simulink model "TST_RailP_PRV"  (R2016b)
settings: Solver=FixedStepDiscrete  StartTime=0.0  StopTime=simTime  FixedStep=sampleTime  RelTol=1e-3
values from neighbouring files (symbols this model uses):
  testCase = 1    [initTST_RailP_PRV_001.m]    (also in initTST_RailP_PRV_002.m = 2)
libraries: UnitTest_Lib x18, simulink x3
settings Model: Creator=liangyunbo  LastModifiedBy=liangyunbo
settings DebuggingCC: SignalRangeChecking=error

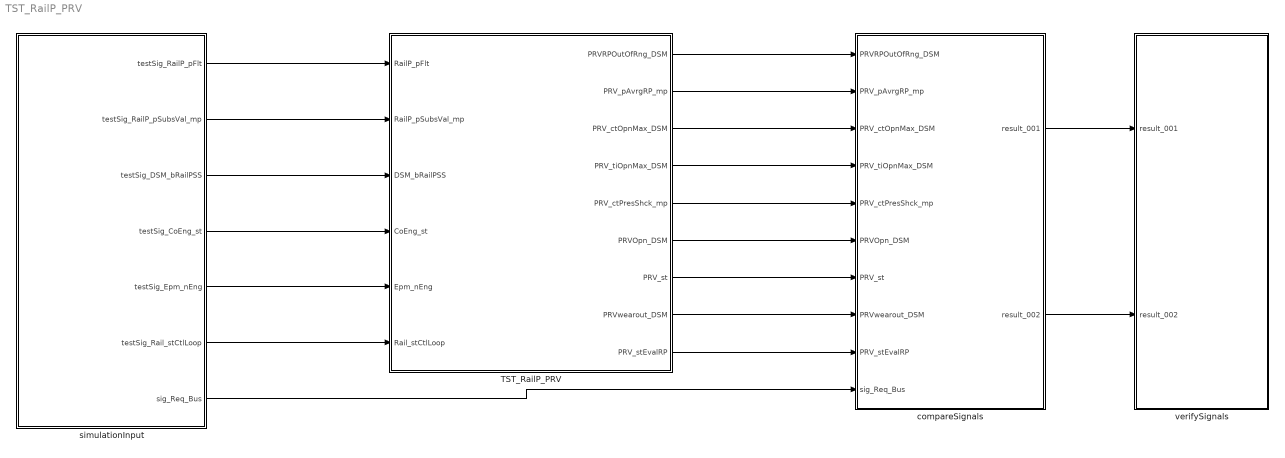
== system TST_RailP_PRV ==
  TST_RailP_PRV : Subsystem
  compareSignals : Subsystem
  simulationInput : Subsystem
  verifySignals : Subsystem
  wires:
  simulationInput/1(testSig_RailP_pFlt) -> TST_RailP_PRV/1(RailP_pFlt)
  simulationInput/2(testSig_RailP_pSubsVal_mp) -> TST_RailP_PRV/2(RailP_pSubsVal_mp)
  simulationInput/3(testSig_DSM_bRailPSS) -> TST_RailP_PRV/3(DSM_bRailPSS)
  simulationInput/4(testSig_CoEng_st) -> TST_RailP_PRV/4(CoEng_st)
  simulationInput/5(testSig_Epm_nEng) -> TST_RailP_PRV/5(Epm_nEng)
  simulationInput/6(testSig_Rail_stCtlLoop) -> TST_RailP_PRV/6(Rail_stCtlLoop)
  TST_RailP_PRV/1(PRVRPOutOfRng_DSM) -> compareSignals/1(PRVRPOutOfRng_DSM)
  TST_RailP_PRV/2(PRV_pAvrgRP_mp) -> compareSignals/2(PRV_pAvrgRP_mp)
  TST_RailP_PRV/3(PRV_ctOpnMax_DSM) -> compareSignals/3(PRV_ctOpnMax_DSM)
  TST_RailP_PRV/4(PRV_tiOpnMax_DSM) -> compareSignals/4(PRV_tiOpnMax_DSM)
  TST_RailP_PRV/5(PRV_ctPresShck_mp) -> compareSignals/5(PRV_ctPresShck_mp)
  TST_RailP_PRV/6(PRVOpn_DSM) -> compareSignals/6(PRVOpn_DSM)
  TST_RailP_PRV/7(PRV_st) -> compareSignals/7(PRV_st)
  TST_RailP_PRV/8(PRVwearout_DSM) -> compareSignals/8(PRVwearout_DSM)
  TST_RailP_PRV/9(PRV_stEvalRP) -> compareSignals/9(PRV_stEvalRP)
  simulationInput/7(sig_Req_Bus) -> compareSignals/10(sig_Req_Bus)
  compareSignals/1(result_001) -> verifySignals/1(result_001)
  compareSignals/2(result_002) -> verifySignals/2(result_002)

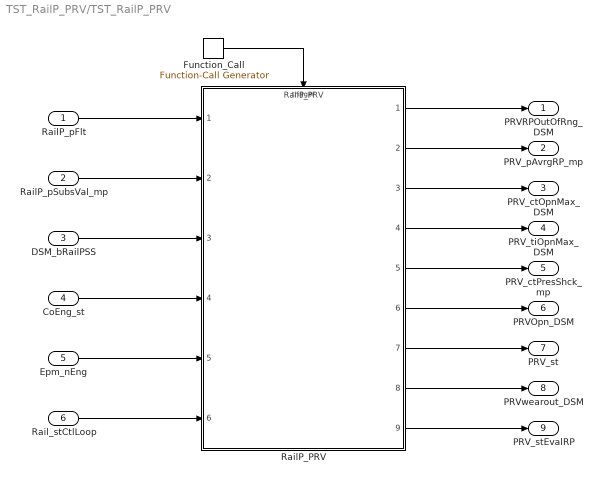
== system TST_RailP_PRV/TST_RailP_PRV ==
  RailP_pFlt : Inport
  RailP_pSubsVal_mp : Inport  Port=2
  DSM_bRailPSS : Inport  Port=3
  CoEng_st : Inport  Port=4
  Epm_nEng : Inport  Port=5
  Rail_stCtlLoop : Inport  Port=6
  Function_Call : simulink/Ports & Subsystems/Function-Call Generator  sample_time=sampleTime  numberOfIterations=1
  RailP_PRV : ModelReference  ModelNameDialog=RailP_PRV  SimulationMode=Normal  ModelReferenceVersion=1.208  TriggerPortName=function  TriggerPortTriggerType=function-call  TriggerPortStatesWhenEnabling=held
  PRVRPOutOfRng_DSM : Outport
  PRV_pAvrgRP_mp : Outport  Port=2
  PRV_ctOpnMax_DSM : Outport  Port=3
  PRV_tiOpnMax_DSM : Outport  Port=4
  PRV_ctPresShck_mp : Outport  Port=5
  PRVOpn_DSM : Outport  Port=6
  PRV_st : Outport  Port=7
  PRVwearout_DSM : Outport  Port=8
  PRV_stEvalRP : Outport  Port=9
  wires:
  Function_Call/1 -> RailP_PRV/Trigger
  RailP_pFlt/1 -> RailP_PRV/1
  RailP_pSubsVal_mp/1 -> RailP_PRV/2
  DSM_bRailPSS/1 -> RailP_PRV/3
  CoEng_st/1 -> RailP_PRV/4
  Epm_nEng/1 -> RailP_PRV/5
  Rail_stCtlLoop/1 -> RailP_PRV/6
  RailP_PRV/1 -> PRVRPOutOfRng_DSM/1
  RailP_PRV/2 -> PRV_pAvrgRP_mp/1
  RailP_PRV/3 -> PRV_ctOpnMax_DSM/1
  RailP_PRV/4 -> PRV_tiOpnMax_DSM/1
  RailP_PRV/5 -> PRV_ctPresShck_mp/1
  RailP_PRV/6 -> PRVOpn_DSM/1
  RailP_PRV/7 -> PRV_st/1
  RailP_PRV/8 -> PRVwearout_DSM/1
  RailP_PRV/9 -> PRV_stEvalRP/1

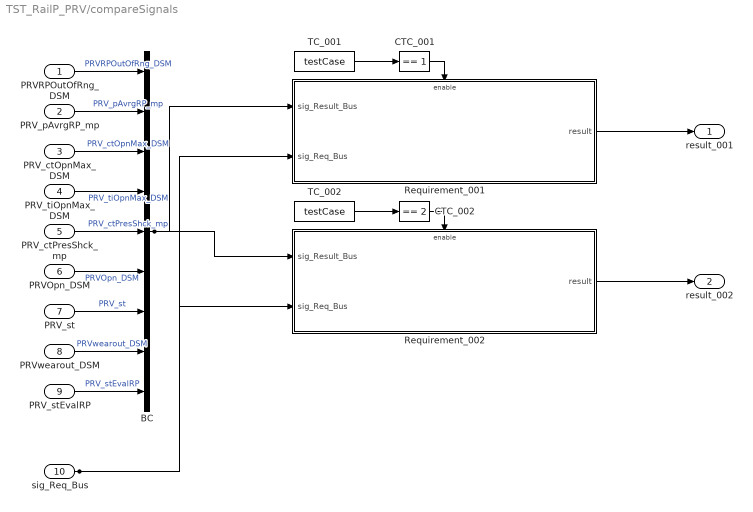
== system TST_RailP_PRV/compareSignals ==
  PRVRPOutOfRng_DSM : Inport
  PRV_pAvrgRP_mp : Inport  Port=2
  PRV_ctOpnMax_DSM : Inport  Port=3
  PRV_tiOpnMax_DSM : Inport  Port=4
  PRV_ctPresShck_mp : Inport  Port=5
  PRVOpn_DSM : Inport  Port=6
  PRV_st : Inport  Port=7
  PRVwearout_DSM : Inport  Port=8
  PRV_stEvalRP : Inport  Port=9
  sig_Req_Bus : Inport  Port=10
  BC : BusCreator  Inputs=9
  CTC_001 : simulink/Logic and Bit Operations/Compare To Constant  relop===  const=1  OutDataTypeStr=boolean
  CTC_002 : simulink/Logic and Bit Operations/Compare To Constant  relop===  const=2  OutDataTypeStr=boolean
  Requirement_001 : Subsystem
  Requirement_002 : Subsystem
  TC_001 : Constant  Value=testCase
  TC_002 : Constant  Value=testCase
  result_001 : Outport
  result_002 : Outport  Port=2
  wires:
  PRVRPOutOfRng_DSM/1 -> BC/1  "PRVRPOutOfRng_DSM"
  PRV_pAvrgRP_mp/1 -> BC/2  "PRV_pAvrgRP_mp"
  PRV_ctOpnMax_DSM/1 -> BC/3  "PRV_ctOpnMax_DSM"
  PRV_tiOpnMax_DSM/1 -> BC/4  "PRV_tiOpnMax_DSM"
  PRV_ctPresShck_mp/1 -> BC/5  "PRV_ctPresShck_mp"
  PRVOpn_DSM/1 -> BC/6  "PRVOpn_DSM"
  PRV_st/1 -> BC/7  "PRV_st"
  PRVwearout_DSM/1 -> BC/8  "PRVwearout_DSM"
  PRV_stEvalRP/1 -> BC/9  "PRV_stEvalRP"
  TC_001/1 -> CTC_001/1
  CTC_001/1 -> Requirement_001/Enable
  sig_Req_Bus/1 -> Requirement_001/2(sig_Req_Bus), Requirement_002/2(sig_Req_Bus)
  BC/1 -> Requirement_001/1(sig_Result_Bus), Requirement_002/1(sig_Result_Bus)
  Requirement_001/1(result) -> result_001/1
  TC_002/1 -> CTC_002/1
  CTC_002/1 -> Requirement_002/Enable
  Requirement_002/1(result) -> result_002/1

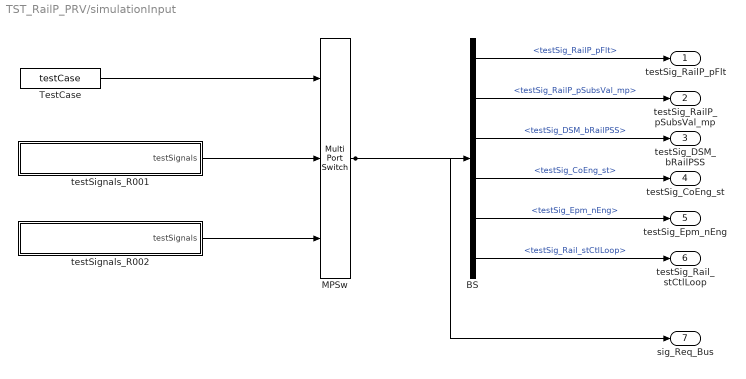
== system TST_RailP_PRV/simulationInput ==
  BS : BusSelector  OutputSignals=testSig_RailP_pFlt,testSig_RailP_pSubsVal_mp,testSig_DSM_bRailPSS,testSig_CoEng_st,testSig_Epm_nEng,testSig_Rail_stCtlLoop
  MPSw : MultiPortSwitch  Inputs=2  SaturateOnIntegerOverflow=on  InputSameDT=on
  TestCase : Constant  Value=testCase
  testSignals_R001 : Subsystem
  testSignals_R002 : Subsystem
  testSig_RailP_pFlt : Outport
  testSig_RailP_pSubsVal_mp : Outport  Port=2
  testSig_DSM_bRailPSS : Outport  Port=3
  testSig_CoEng_st : Outport  Port=4
  testSig_Epm_nEng : Outport  Port=5
  testSig_Rail_stCtlLoop : Outport  Port=6
  sig_Req_Bus : Outport  Port=7
  wires:
  BS/1 -> testSig_RailP_pFlt/1  "<testSig_RailP_pFlt>"
  BS/2 -> testSig_RailP_pSubsVal_mp/1  "<testSig_RailP_pSubsVal_mp>"
  BS/3 -> testSig_DSM_bRailPSS/1  "<testSig_DSM_bRailPSS>"
  BS/4 -> testSig_CoEng_st/1  "<testSig_CoEng_st>"
  BS/5 -> testSig_Epm_nEng/1  "<testSig_Epm_nEng>"
  BS/6 -> testSig_Rail_stCtlLoop/1  "<testSig_Rail_stCtlLoop>"
  MPSw/1 -> BS/1, sig_Req_Bus/1
  TestCase/1 -> MPSw/1
  testSignals_R001/1(testSignals) -> MPSw/2
  testSignals_R002/1(testSignals) -> MPSw/3

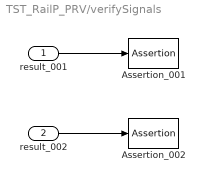
== system TST_RailP_PRV/verifySignals ==
  result_001 : Inport
  result_002 : Inport  Port=2
  Assertion_001 : Assertion  Enabled=off
  Assertion_002 : Assertion  Enabled=off
  wires:
  result_001/1 -> Assertion_001/1
  result_002/1 -> Assertion_002/1

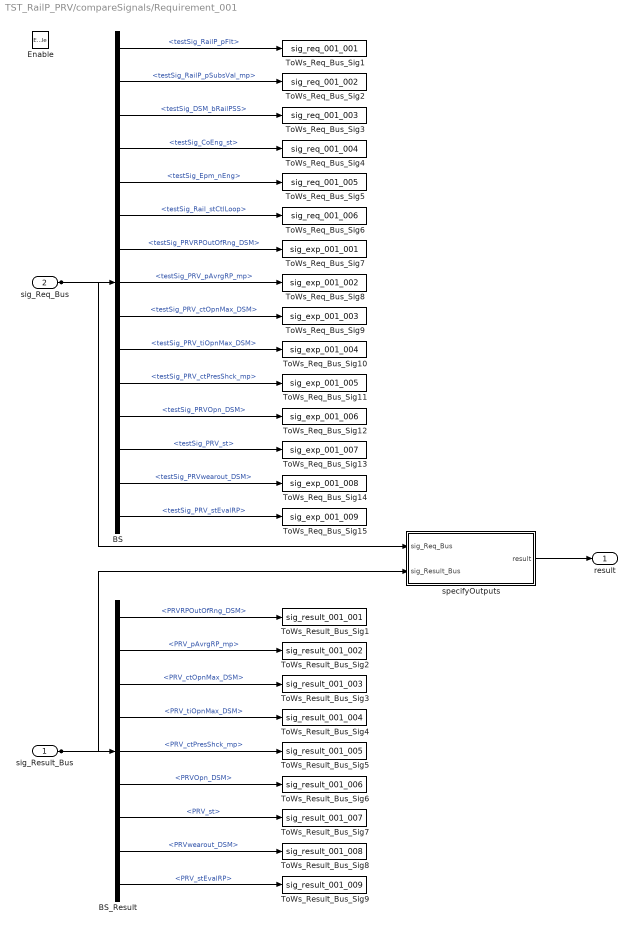
== system TST_RailP_PRV/compareSignals/Requirement_001 ==
  sig_Result_Bus : Inport
  sig_Req_Bus : Inport  Port=2
  Enable : EnablePort
  BS : BusSelector  OutputSignals=testSig_RailP_pFlt,testSig_RailP_pSubsVal_mp,testSig_DSM_bRailPSS,testSig_CoEng_st,testSig_Epm_nEng,testSig_Rail_stCtlLoop,testSig_PRVRPOutOfRng_DSM,testSig_PRV_pAvrgRP_mp,testSig_PRV_ctOpnMax_DSM,testSig_PRV_tiOpnMax_DSM,testSig_PRV_ctPresShck_mp,testSig_PRVOpn_DSM,testSig_PRV_st,testSig_PRVwearout_DSM,testSig_PRV_stEvalRP
  BS_Result : BusSelector  OutputSignals=PRVRPOutOfRng_DSM,PRV_pAvrgRP_mp,PRV_ctOpnMax_DSM,PRV_tiOpnMax_DSM,PRV_ctPresShck_mp,PRVOpn_DSM,PRV_st,PRVwearout_DSM,PRV_stEvalRP
  ToWs_Req_Bus_Sig1 : ToWorkspace  VariableName=sig_req_001_001  SaveFormat=Structure With Time
  ToWs_Req_Bus_Sig10 : ToWorkspace  VariableName=sig_exp_001_004  SaveFormat=Structure With Time
  ToWs_Req_Bus_Sig11 : ToWorkspace  VariableName=sig_exp_001_005  SaveFormat=Structure With Time
  ToWs_Req_Bus_Sig12 : ToWorkspace  VariableName=sig_exp_001_006  SaveFormat=Structure With Time
  ToWs_Req_Bus_Sig13 : ToWorkspace  VariableName=sig_exp_001_007  SaveFormat=Structure With Time
  ToWs_Req_Bus_Sig14 : ToWorkspace  VariableName=sig_exp_001_008  SaveFormat=Structure With Time
  ToWs_Req_Bus_Sig15 : ToWorkspace  VariableName=sig_exp_001_009  SaveFormat=Structure With Time
  ToWs_Req_Bus_Sig2 : ToWorkspace  VariableName=sig_req_001_002  SaveFormat=Structure With Time
  ToWs_Req_Bus_Sig3 : ToWorkspace  VariableName=sig_req_001_003  SaveFormat=Structure With Time
  ToWs_Req_Bus_Sig4 : ToWorkspace  VariableName=sig_req_001_004  SaveFormat=Structure With Time
  ToWs_Req_Bus_Sig5 : ToWorkspace  VariableName=sig_req_001_005  SaveFormat=Structure With Time
  ToWs_Req_Bus_Sig6 : ToWorkspace  VariableName=sig_req_001_006  SaveFormat=Structure With Time
  ToWs_Req_Bus_Sig7 : ToWorkspace  VariableName=sig_exp_001_001  SaveFormat=Structure With Time
  ToWs_Req_Bus_Sig8 : ToWorkspace  VariableName=sig_exp_001_002  SaveFormat=Structure With Time
  ToWs_Req_Bus_Sig9 : ToWorkspace  VariableName=sig_exp_001_003  SaveFormat=Structure With Time
  ToWs_Result_Bus_Sig1 : ToWorkspace  VariableName=sig_result_001_001  SaveFormat=Structure With Time
  ToWs_Result_Bus_Sig2 : ToWorkspace  VariableName=sig_result_001_002  SaveFormat=Structure With Time
  ToWs_Result_Bus_Sig3 : ToWorkspace  VariableName=sig_result_001_003  SaveFormat=Structure With Time
  ToWs_Result_Bus_Sig4 : ToWorkspace  VariableName=sig_result_001_004  SaveFormat=Structure With Time
  ToWs_Result_Bus_Sig5 : ToWorkspace  VariableName=sig_result_001_005  SaveFormat=Structure With Time
  ToWs_Result_Bus_Sig6 : ToWorkspace  VariableName=sig_result_001_006  SaveFormat=Structure With Time
  ToWs_Result_Bus_Sig7 : ToWorkspace  VariableName=sig_result_001_007  SaveFormat=Structure With Time
  ToWs_Result_Bus_Sig8 : ToWorkspace  VariableName=sig_result_001_008  SaveFormat=Structure With Time
  ToWs_Result_Bus_Sig9 : ToWorkspace  VariableName=sig_result_001_009  SaveFormat=Structure With Time
  specifyOutputs : Subsystem
  result : Outport
  wires:
  sig_Req_Bus/1 -> BS/1, specifyOutputs/1(sig_Req_Bus)
  BS/1 -> ToWs_Req_Bus_Sig1/1  "<testSig_RailP_pFlt>"
  BS/2 -> ToWs_Req_Bus_Sig2/1  "<testSig_RailP_pSubsVal_mp>"
  BS/3 -> ToWs_Req_Bus_Sig3/1  "<testSig_DSM_bRailPSS>"
  BS/4 -> ToWs_Req_Bus_Sig4/1  "<testSig_CoEng_st>"
  BS/5 -> ToWs_Req_Bus_Sig5/1  "<testSig_Epm_nEng>"
  BS/6 -> ToWs_Req_Bus_Sig6/1  "<testSig_Rail_stCtlLoop>"
  BS/7 -> ToWs_Req_Bus_Sig7/1  "<testSig_PRVRPOutOfRng_DSM>"
  BS/8 -> ToWs_Req_Bus_Sig8/1  "<testSig_PRV_pAvrgRP_mp>"
  BS/9 -> ToWs_Req_Bus_Sig9/1  "<testSig_PRV_ctOpnMax_DSM>"
  BS/10 -> ToWs_Req_Bus_Sig10/1  "<testSig_PRV_tiOpnMax_DSM>"
  BS/11 -> ToWs_Req_Bus_Sig11/1  "<testSig_PRV_ctPresShck_mp>"
  BS/12 -> ToWs_Req_Bus_Sig12/1  "<testSig_PRVOpn_DSM>"
  BS/13 -> ToWs_Req_Bus_Sig13/1  "<testSig_PRV_st>"
  BS/14 -> ToWs_Req_Bus_Sig14/1  "<testSig_PRVwearout_DSM>"
  BS/15 -> ToWs_Req_Bus_Sig15/1  "<testSig_PRV_stEvalRP>"
  sig_Result_Bus/1 -> BS_Result/1, specifyOutputs/2(sig_Result_Bus)
  BS_Result/1 -> ToWs_Result_Bus_Sig1/1  "<PRVRPOutOfRng_DSM>"
  BS_Result/2 -> ToWs_Result_Bus_Sig2/1  "<PRV_pAvrgRP_mp>"
  BS_Result/3 -> ToWs_Result_Bus_Sig3/1  "<PRV_ctOpnMax_DSM>"
  BS_Result/4 -> ToWs_Result_Bus_Sig4/1  "<PRV_tiOpnMax_DSM>"
  BS_Result/5 -> ToWs_Result_Bus_Sig5/1  "<PRV_ctPresShck_mp>"
  BS_Result/6 -> ToWs_Result_Bus_Sig6/1  "<PRVOpn_DSM>"
  BS_Result/7 -> ToWs_Result_Bus_Sig7/1  "<PRV_st>"
  BS_Result/8 -> ToWs_Result_Bus_Sig8/1  "<PRVwearout_DSM>"
  BS_Result/9 -> ToWs_Result_Bus_Sig9/1  "<PRV_stEvalRP>"
  specifyOutputs/1(result) -> result/1

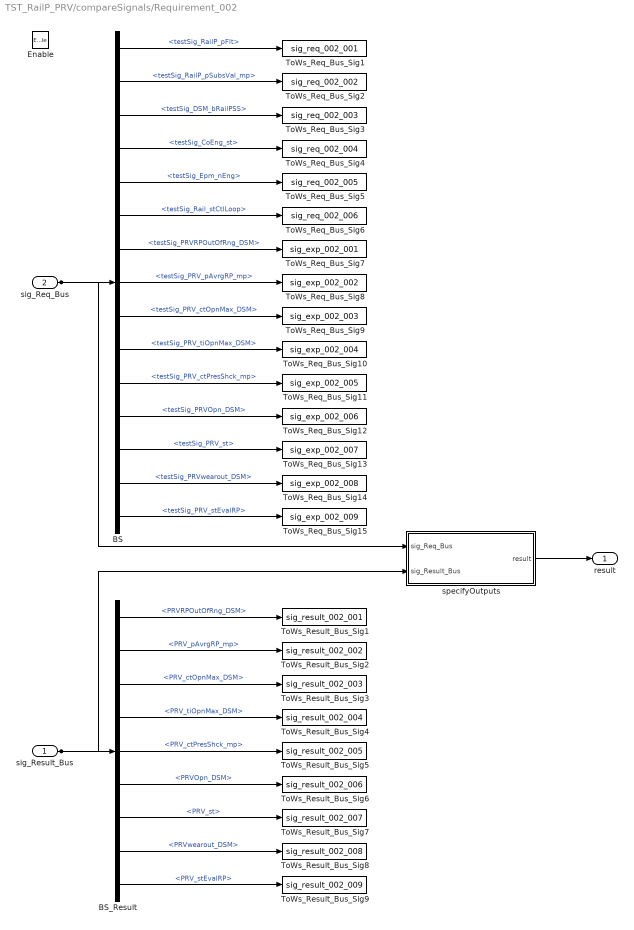
== system TST_RailP_PRV/compareSignals/Requirement_002 ==
  sig_Result_Bus : Inport
  sig_Req_Bus : Inport  Port=2
  Enable : EnablePort
  BS : BusSelector  OutputSignals=testSig_RailP_pFlt,testSig_RailP_pSubsVal_mp,testSig_DSM_bRailPSS,testSig_CoEng_st,testSig_Epm_nEng,testSig_Rail_stCtlLoop,testSig_PRVRPOutOfRng_DSM,testSig_PRV_pAvrgRP_mp,testSig_PRV_ctOpnMax_DSM,testSig_PRV_tiOpnMax_DSM,testSig_PRV_ctPresShck_mp,testSig_PRVOpn_DSM,testSig_PRV_st,testSig_PRVwearout_DSM,testSig_PRV_stEvalRP
  BS_Result : BusSelector  OutputSignals=PRVRPOutOfRng_DSM,PRV_pAvrgRP_mp,PRV_ctOpnMax_DSM,PRV_tiOpnMax_DSM,PRV_ctPresShck_mp,PRVOpn_DSM,PRV_st,PRVwearout_DSM,PRV_stEvalRP
  ToWs_Req_Bus_Sig1 : ToWorkspace  VariableName=sig_req_002_001  SaveFormat=Structure With Time
  ToWs_Req_Bus_Sig10 : ToWorkspace  VariableName=sig_exp_002_004  SaveFormat=Structure With Time
  ToWs_Req_Bus_Sig11 : ToWorkspace  VariableName=sig_exp_002_005  SaveFormat=Structure With Time
  ToWs_Req_Bus_Sig12 : ToWorkspace  VariableName=sig_exp_002_006  SaveFormat=Structure With Time
  ToWs_Req_Bus_Sig13 : ToWorkspace  VariableName=sig_exp_002_007  SaveFormat=Structure With Time
  ToWs_Req_Bus_Sig14 : ToWorkspace  VariableName=sig_exp_002_008  SaveFormat=Structure With Time
  ToWs_Req_Bus_Sig15 : ToWorkspace  VariableName=sig_exp_002_009  SaveFormat=Structure With Time
  ToWs_Req_Bus_Sig2 : ToWorkspace  VariableName=sig_req_002_002  SaveFormat=Structure With Time
  ToWs_Req_Bus_Sig3 : ToWorkspace  VariableName=sig_req_002_003  SaveFormat=Structure With Time
  ToWs_Req_Bus_Sig4 : ToWorkspace  VariableName=sig_req_002_004  SaveFormat=Structure With Time
  ToWs_Req_Bus_Sig5 : ToWorkspace  VariableName=sig_req_002_005  SaveFormat=Structure With Time
  ToWs_Req_Bus_Sig6 : ToWorkspace  VariableName=sig_req_002_006  SaveFormat=Structure With Time
  ToWs_Req_Bus_Sig7 : ToWorkspace  VariableName=sig_exp_002_001  SaveFormat=Structure With Time
  ToWs_Req_Bus_Sig8 : ToWorkspace  VariableName=sig_exp_002_002  SaveFormat=Structure With Time
  ToWs_Req_Bus_Sig9 : ToWorkspace  VariableName=sig_exp_002_003  SaveFormat=Structure With Time
  ToWs_Result_Bus_Sig1 : ToWorkspace  VariableName=sig_result_002_001  SaveFormat=Structure With Time
  ToWs_Result_Bus_Sig2 : ToWorkspace  VariableName=sig_result_002_002  SaveFormat=Structure With Time
  ToWs_Result_Bus_Sig3 : ToWorkspace  VariableName=sig_result_002_003  SaveFormat=Structure With Time
  ToWs_Result_Bus_Sig4 : ToWorkspace  VariableName=sig_result_002_004  SaveFormat=Structure With Time
  ToWs_Result_Bus_Sig5 : ToWorkspace  VariableName=sig_result_002_005  SaveFormat=Structure With Time
  ToWs_Result_Bus_Sig6 : ToWorkspace  VariableName=sig_result_002_006  SaveFormat=Structure With Time
  ToWs_Result_Bus_Sig7 : ToWorkspace  VariableName=sig_result_002_007  SaveFormat=Structure With Time
  ToWs_Result_Bus_Sig8 : ToWorkspace  VariableName=sig_result_002_008  SaveFormat=Structure With Time
  ToWs_Result_Bus_Sig9 : ToWorkspace  VariableName=sig_result_002_009  SaveFormat=Structure With Time
  specifyOutputs : Subsystem
  result : Outport
  wires:
  sig_Req_Bus/1 -> BS/1, specifyOutputs/1(sig_Req_Bus)
  BS/1 -> ToWs_Req_Bus_Sig1/1  "<testSig_RailP_pFlt>"
  BS/2 -> ToWs_Req_Bus_Sig2/1  "<testSig_RailP_pSubsVal_mp>"
  BS/3 -> ToWs_Req_Bus_Sig3/1  "<testSig_DSM_bRailPSS>"
  BS/4 -> ToWs_Req_Bus_Sig4/1  "<testSig_CoEng_st>"
  BS/5 -> ToWs_Req_Bus_Sig5/1  "<testSig_Epm_nEng>"
  BS/6 -> ToWs_Req_Bus_Sig6/1  "<testSig_Rail_stCtlLoop>"
  BS/7 -> ToWs_Req_Bus_Sig7/1  "<testSig_PRVRPOutOfRng_DSM>"
  BS/8 -> ToWs_Req_Bus_Sig8/1  "<testSig_PRV_pAvrgRP_mp>"
  BS/9 -> ToWs_Req_Bus_Sig9/1  "<testSig_PRV_ctOpnMax_DSM>"
  BS/10 -> ToWs_Req_Bus_Sig10/1  "<testSig_PRV_tiOpnMax_DSM>"
  BS/11 -> ToWs_Req_Bus_Sig11/1  "<testSig_PRV_ctPresShck_mp>"
  BS/12 -> ToWs_Req_Bus_Sig12/1  "<testSig_PRVOpn_DSM>"
  BS/13 -> ToWs_Req_Bus_Sig13/1  "<testSig_PRV_st>"
  BS/14 -> ToWs_Req_Bus_Sig14/1  "<testSig_PRVwearout_DSM>"
  BS/15 -> ToWs_Req_Bus_Sig15/1  "<testSig_PRV_stEvalRP>"
  sig_Result_Bus/1 -> BS_Result/1, specifyOutputs/2(sig_Result_Bus)
  BS_Result/1 -> ToWs_Result_Bus_Sig1/1  "<PRVRPOutOfRng_DSM>"
  BS_Result/2 -> ToWs_Result_Bus_Sig2/1  "<PRV_pAvrgRP_mp>"
  BS_Result/3 -> ToWs_Result_Bus_Sig3/1  "<PRV_ctOpnMax_DSM>"
  BS_Result/4 -> ToWs_Result_Bus_Sig4/1  "<PRV_tiOpnMax_DSM>"
  BS_Result/5 -> ToWs_Result_Bus_Sig5/1  "<PRV_ctPresShck_mp>"
  BS_Result/6 -> ToWs_Result_Bus_Sig6/1  "<PRVOpn_DSM>"
  BS_Result/7 -> ToWs_Result_Bus_Sig7/1  "<PRV_st>"
  BS_Result/8 -> ToWs_Result_Bus_Sig8/1  "<PRVwearout_DSM>"
  BS_Result/9 -> ToWs_Result_Bus_Sig9/1  "<PRV_stEvalRP>"
  specifyOutputs/1(result) -> result/1

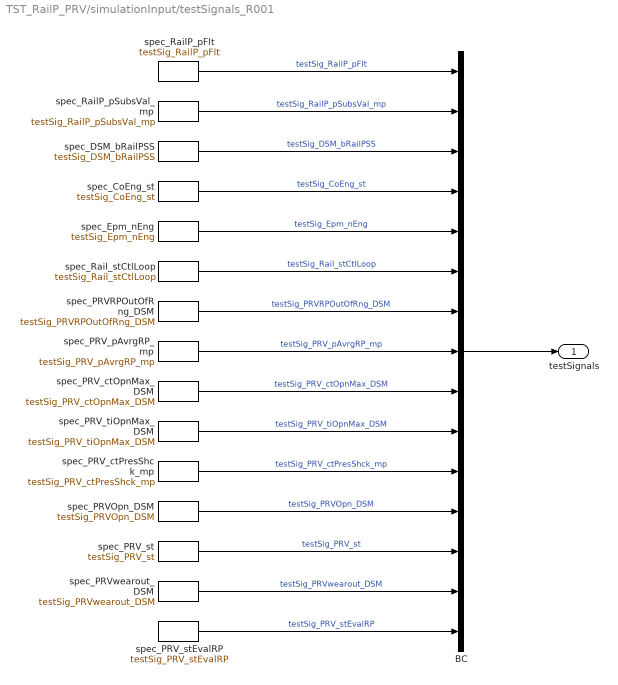
== system TST_RailP_PRV/simulationInput/testSignals_R001 ==
  BC : BusCreator  Inputs=15
  spec_CoEng_st : FromWorkspace  VariableName=testSig_CoEng_st  Interpolate=off  OutputAfterFinalValue=Holding final value
  spec_DSM_bRailPSS : FromWorkspace  VariableName=testSig_DSM_bRailPSS  Interpolate=off  OutputAfterFinalValue=Holding final value
  spec_Epm_nEng : FromWorkspace  VariableName=testSig_Epm_nEng  Interpolate=off  OutputAfterFinalValue=Holding final value
  spec_PRVOpn_DSM : FromWorkspace  VariableName=testSig_PRVOpn_DSM  Interpolate=off  OutputAfterFinalValue=Holding final value
  spec_PRVRPOutOfRng_DSM : FromWorkspace  VariableName=testSig_PRVRPOutOfRng_DSM  Interpolate=off  OutputAfterFinalValue=Holding final value
  spec_PRV_ctOpnMax_DSM : FromWorkspace  VariableName=testSig_PRV_ctOpnMax_DSM  Interpolate=off  OutputAfterFinalValue=Holding final value
  spec_PRV_ctPresShck_mp : FromWorkspace  VariableName=testSig_PRV_ctPresShck_mp  Interpolate=off  OutputAfterFinalValue=Holding final value
  spec_PRV_pAvrgRP_mp : FromWorkspace  VariableName=testSig_PRV_pAvrgRP_mp  Interpolate=off  OutputAfterFinalValue=Holding final value
  spec_PRV_st : FromWorkspace  VariableName=testSig_PRV_st  Interpolate=off  OutputAfterFinalValue=Holding final value
  spec_PRV_stEvalRP : FromWorkspace  VariableName=testSig_PRV_stEvalRP  Interpolate=off  OutputAfterFinalValue=Holding final value
  spec_PRV_tiOpnMax_DSM : FromWorkspace  VariableName=testSig_PRV_tiOpnMax_DSM  Interpolate=off  OutputAfterFinalValue=Holding final value
  spec_PRVwearout_DSM : FromWorkspace  VariableName=testSig_PRVwearout_DSM  Interpolate=off  OutputAfterFinalValue=Holding final value
  spec_RailP_pFlt : FromWorkspace  VariableName=testSig_RailP_pFlt  Interpolate=off  OutputAfterFinalValue=Holding final value
  spec_RailP_pSubsVal_mp : FromWorkspace  VariableName=testSig_RailP_pSubsVal_mp  Interpolate=off  OutputAfterFinalValue=Holding final value
  spec_Rail_stCtlLoop : FromWorkspace  VariableName=testSig_Rail_stCtlLoop  Interpolate=off  OutputAfterFinalValue=Holding final value
  testSignals : Outport
  wires:
  BC/1 -> testSignals/1
  spec_RailP_pFlt/1 -> BC/1  "testSig_RailP_pFlt"
  spec_RailP_pSubsVal_mp/1 -> BC/2  "testSig_RailP_pSubsVal_mp"
  spec_DSM_bRailPSS/1 -> BC/3  "testSig_DSM_bRailPSS"
  spec_CoEng_st/1 -> BC/4  "testSig_CoEng_st"
  spec_Epm_nEng/1 -> BC/5  "testSig_Epm_nEng"
  spec_Rail_stCtlLoop/1 -> BC/6  "testSig_Rail_stCtlLoop"
  spec_PRVRPOutOfRng_DSM/1 -> BC/7  "testSig_PRVRPOutOfRng_DSM"
  spec_PRV_pAvrgRP_mp/1 -> BC/8  "testSig_PRV_pAvrgRP_mp"
  spec_PRV_ctOpnMax_DSM/1 -> BC/9  "testSig_PRV_ctOpnMax_DSM"
  spec_PRV_tiOpnMax_DSM/1 -> BC/10  "testSig_PRV_tiOpnMax_DSM"
  spec_PRV_ctPresShck_mp/1 -> BC/11  "testSig_PRV_ctPresShck_mp"
  spec_PRVOpn_DSM/1 -> BC/12  "testSig_PRVOpn_DSM"
  spec_PRV_st/1 -> BC/13  "testSig_PRV_st"
  spec_PRVwearout_DSM/1 -> BC/14  "testSig_PRVwearout_DSM"
  spec_PRV_stEvalRP/1 -> BC/15  "testSig_PRV_stEvalRP"

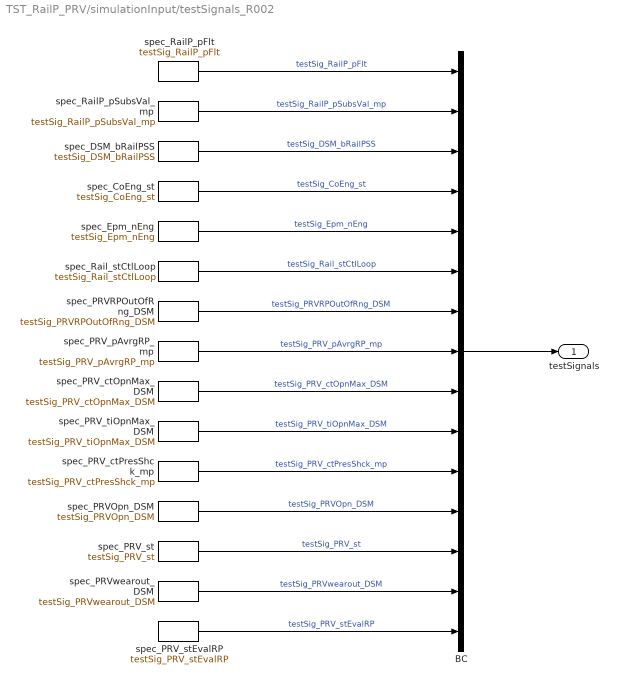
== system TST_RailP_PRV/simulationInput/testSignals_R002 ==
  BC : BusCreator  Inputs=15
  spec_CoEng_st : FromWorkspace  VariableName=testSig_CoEng_st  Interpolate=off  OutputAfterFinalValue=Holding final value
  spec_DSM_bRailPSS : FromWorkspace  VariableName=testSig_DSM_bRailPSS  Interpolate=off  OutputAfterFinalValue=Holding final value
  spec_Epm_nEng : FromWorkspace  VariableName=testSig_Epm_nEng  Interpolate=off  OutputAfterFinalValue=Holding final value
  spec_PRVOpn_DSM : FromWorkspace  VariableName=testSig_PRVOpn_DSM  Interpolate=off  OutputAfterFinalValue=Holding final value
  spec_PRVRPOutOfRng_DSM : FromWorkspace  VariableName=testSig_PRVRPOutOfRng_DSM  Interpolate=off  OutputAfterFinalValue=Holding final value
  spec_PRV_ctOpnMax_DSM : FromWorkspace  VariableName=testSig_PRV_ctOpnMax_DSM  Interpolate=off  OutputAfterFinalValue=Holding final value
  spec_PRV_ctPresShck_mp : FromWorkspace  VariableName=testSig_PRV_ctPresShck_mp  Interpolate=off  OutputAfterFinalValue=Holding final value
  spec_PRV_pAvrgRP_mp : FromWorkspace  VariableName=testSig_PRV_pAvrgRP_mp  Interpolate=off  OutputAfterFinalValue=Holding final value
  spec_PRV_st : FromWorkspace  VariableName=testSig_PRV_st  Interpolate=off  OutputAfterFinalValue=Holding final value
  spec_PRV_stEvalRP : FromWorkspace  VariableName=testSig_PRV_stEvalRP  Interpolate=off  OutputAfterFinalValue=Holding final value
  spec_PRV_tiOpnMax_DSM : FromWorkspace  VariableName=testSig_PRV_tiOpnMax_DSM  Interpolate=off  OutputAfterFinalValue=Holding final value
  spec_PRVwearout_DSM : FromWorkspace  VariableName=testSig_PRVwearout_DSM  Interpolate=off  OutputAfterFinalValue=Holding final value
  spec_RailP_pFlt : FromWorkspace  VariableName=testSig_RailP_pFlt  Interpolate=off  OutputAfterFinalValue=Holding final value
  spec_RailP_pSubsVal_mp : FromWorkspace  VariableName=testSig_RailP_pSubsVal_mp  Interpolate=off  OutputAfterFinalValue=Holding final value
  spec_Rail_stCtlLoop : FromWorkspace  VariableName=testSig_Rail_stCtlLoop  Interpolate=off  OutputAfterFinalValue=Holding final value
  testSignals : Outport
  wires:
  BC/1 -> testSignals/1
  spec_RailP_pFlt/1 -> BC/1  "testSig_RailP_pFlt"
  spec_RailP_pSubsVal_mp/1 -> BC/2  "testSig_RailP_pSubsVal_mp"
  spec_DSM_bRailPSS/1 -> BC/3  "testSig_DSM_bRailPSS"
  spec_CoEng_st/1 -> BC/4  "testSig_CoEng_st"
  spec_Epm_nEng/1 -> BC/5  "testSig_Epm_nEng"
  spec_Rail_stCtlLoop/1 -> BC/6  "testSig_Rail_stCtlLoop"
  spec_PRVRPOutOfRng_DSM/1 -> BC/7  "testSig_PRVRPOutOfRng_DSM"
  spec_PRV_pAvrgRP_mp/1 -> BC/8  "testSig_PRV_pAvrgRP_mp"
  spec_PRV_ctOpnMax_DSM/1 -> BC/9  "testSig_PRV_ctOpnMax_DSM"
  spec_PRV_tiOpnMax_DSM/1 -> BC/10  "testSig_PRV_tiOpnMax_DSM"
  spec_PRV_ctPresShck_mp/1 -> BC/11  "testSig_PRV_ctPresShck_mp"
  spec_PRVOpn_DSM/1 -> BC/12  "testSig_PRVOpn_DSM"
  spec_PRV_st/1 -> BC/13  "testSig_PRV_st"
  spec_PRVwearout_DSM/1 -> BC/14  "testSig_PRVwearout_DSM"
  spec_PRV_stEvalRP/1 -> BC/15  "testSig_PRV_stEvalRP"

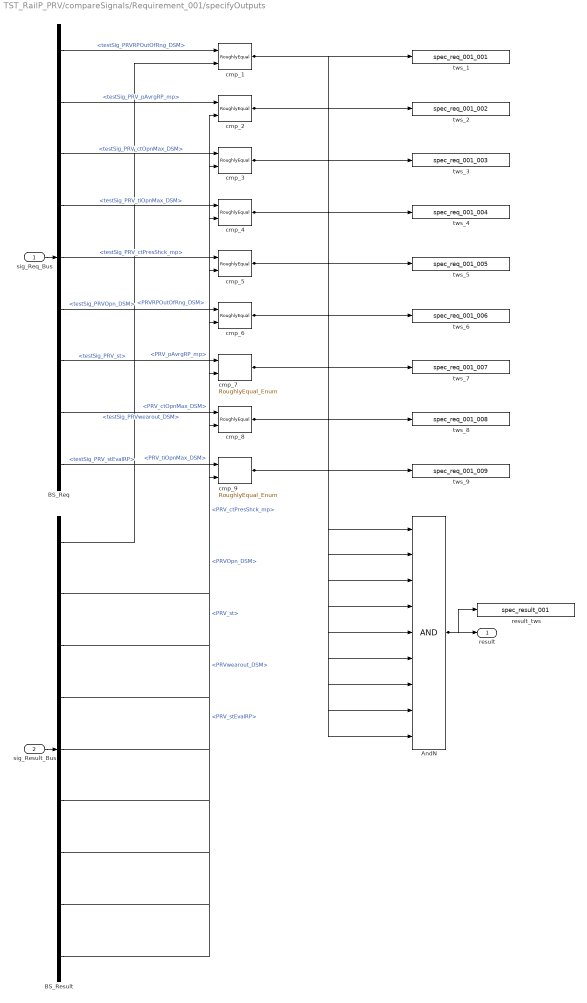
== system TST_RailP_PRV/compareSignals/Requirement_001/specifyOutputs ==
  sig_Req_Bus : Inport
  sig_Result_Bus : Inport  Port=2
  AndN : Logic  Inputs=9
  BS_Req : BusSelector  OutputSignals=testSig_PRVRPOutOfRng_DSM,testSig_PRV_pAvrgRP_mp,testSig_PRV_ctOpnMax_DSM,testSig_PRV_tiOpnMax_DSM,testSig_PRV_ctPresShck_mp,testSig_PRVOpn_DSM,testSig_PRV_st,testSig_PRVwearout_DSM,testSig_PRV_stEvalRP
  BS_Result : BusSelector  OutputSignals=PRVRPOutOfRng_DSM,PRV_pAvrgRP_mp,PRV_ctOpnMax_DSM,PRV_tiOpnMax_DSM,PRV_ctPresShck_mp,PRVOpn_DSM,PRV_st,PRVwearout_DSM,PRV_stEvalRP
  cmp_{1..6,8} (7 alike) : UnitTest_Lib/RoughlyEqual  slope=0.1
  cmp_7 : UnitTest_Lib/RoughlyEqual_Enum  slope=0.1
  cmp_9 : UnitTest_Lib/RoughlyEqual_Enum  slope=0.1
  result_tws : ToWorkspace  VariableName=spec_result_001
  tws_1 : ToWorkspace  VariableName=spec_req_001_001
  tws_2 : ToWorkspace  VariableName=spec_req_001_002
  tws_3 : ToWorkspace  VariableName=spec_req_001_003
  tws_4 : ToWorkspace  VariableName=spec_req_001_004
  tws_5 : ToWorkspace  VariableName=spec_req_001_005
  tws_6 : ToWorkspace  VariableName=spec_req_001_006
  tws_7 : ToWorkspace  VariableName=spec_req_001_007
  tws_8 : ToWorkspace  VariableName=spec_req_001_008
  tws_9 : ToWorkspace  VariableName=spec_req_001_009
  result : Outport
  wires:
  sig_Req_Bus/1 -> BS_Req/1
  sig_Result_Bus/1 -> BS_Result/1
  AndN/1 -> result/1, result_tws/1
  BS_Req/1 -> cmp_1/1  "<testSig_PRVRPOutOfRng_DSM>"
  BS_Result/1 -> cmp_1/2  "<PRVRPOutOfRng_DSM>"
  cmp_1/1 -> tws_1/1, AndN/1
  BS_Req/2 -> cmp_2/1  "<testSig_PRV_pAvrgRP_mp>"
  BS_Result/2 -> cmp_2/2  "<PRV_pAvrgRP_mp>"
  cmp_2/1 -> tws_2/1, AndN/2
  BS_Req/3 -> cmp_3/1  "<testSig_PRV_ctOpnMax_DSM>"
  BS_Result/3 -> cmp_3/2  "<PRV_ctOpnMax_DSM>"
  cmp_3/1 -> tws_3/1, AndN/3
  BS_Req/4 -> cmp_4/1  "<testSig_PRV_tiOpnMax_DSM>"
  BS_Result/4 -> cmp_4/2  "<PRV_tiOpnMax_DSM>"
  cmp_4/1 -> tws_4/1, AndN/4
  BS_Req/5 -> cmp_5/1  "<testSig_PRV_ctPresShck_mp>"
  BS_Result/5 -> cmp_5/2  "<PRV_ctPresShck_mp>"
  cmp_5/1 -> tws_5/1, AndN/5
  BS_Req/6 -> cmp_6/1  "<testSig_PRVOpn_DSM>"
  BS_Result/6 -> cmp_6/2  "<PRVOpn_DSM>"
  cmp_6/1 -> tws_6/1, AndN/6
  BS_Req/7 -> cmp_7/1  "<testSig_PRV_st>"
  BS_Result/7 -> cmp_7/2  "<PRV_st>"
  cmp_7/1 -> tws_7/1, AndN/7
  BS_Req/8 -> cmp_8/1  "<testSig_PRVwearout_DSM>"
  BS_Result/8 -> cmp_8/2  "<PRVwearout_DSM>"
  cmp_8/1 -> tws_8/1, AndN/8
  BS_Req/9 -> cmp_9/1  "<testSig_PRV_stEvalRP>"
  BS_Result/9 -> cmp_9/2  "<PRV_stEvalRP>"
  cmp_9/1 -> tws_9/1, AndN/9

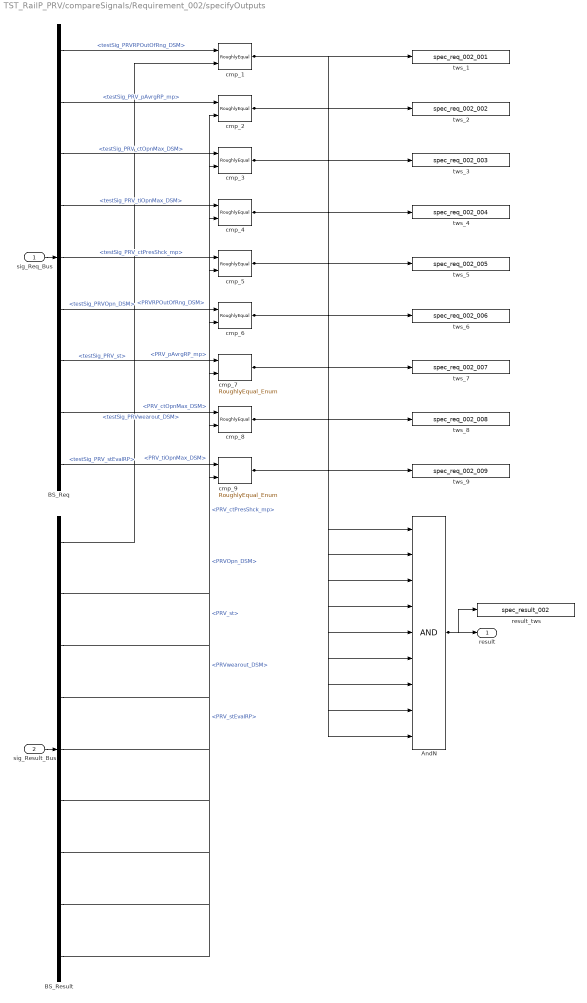
== system TST_RailP_PRV/compareSignals/Requirement_002/specifyOutputs ==
  sig_Req_Bus : Inport
  sig_Result_Bus : Inport  Port=2
  AndN : Logic  Inputs=9
  BS_Req : BusSelector  OutputSignals=testSig_PRVRPOutOfRng_DSM,testSig_PRV_pAvrgRP_mp,testSig_PRV_ctOpnMax_DSM,testSig_PRV_tiOpnMax_DSM,testSig_PRV_ctPresShck_mp,testSig_PRVOpn_DSM,testSig_PRV_st,testSig_PRVwearout_DSM,testSig_PRV_stEvalRP
  BS_Result : BusSelector  OutputSignals=PRVRPOutOfRng_DSM,PRV_pAvrgRP_mp,PRV_ctOpnMax_DSM,PRV_tiOpnMax_DSM,PRV_ctPresShck_mp,PRVOpn_DSM,PRV_st,PRVwearout_DSM,PRV_stEvalRP
  cmp_{1..6,8} (7 alike) : UnitTest_Lib/RoughlyEqual  slope=0.1
  cmp_7 : UnitTest_Lib/RoughlyEqual_Enum  slope=0.1
  cmp_9 : UnitTest_Lib/RoughlyEqual_Enum  slope=0.1
  result_tws : ToWorkspace  VariableName=spec_result_002
  tws_1 : ToWorkspace  VariableName=spec_req_002_001
  tws_2 : ToWorkspace  VariableName=spec_req_002_002
  tws_3 : ToWorkspace  VariableName=spec_req_002_003
  tws_4 : ToWorkspace  VariableName=spec_req_002_004
  tws_5 : ToWorkspace  VariableName=spec_req_002_005
  tws_6 : ToWorkspace  VariableName=spec_req_002_006
  tws_7 : ToWorkspace  VariableName=spec_req_002_007
  tws_8 : ToWorkspace  VariableName=spec_req_002_008
  tws_9 : ToWorkspace  VariableName=spec_req_002_009
  result : Outport
  wires:
  sig_Req_Bus/1 -> BS_Req/1
  sig_Result_Bus/1 -> BS_Result/1
  AndN/1 -> result/1, result_tws/1
  BS_Req/1 -> cmp_1/1  "<testSig_PRVRPOutOfRng_DSM>"
  BS_Result/1 -> cmp_1/2  "<PRVRPOutOfRng_DSM>"
  cmp_1/1 -> tws_1/1, AndN/1
  BS_Req/2 -> cmp_2/1  "<testSig_PRV_pAvrgRP_mp>"
  BS_Result/2 -> cmp_2/2  "<PRV_pAvrgRP_mp>"
  cmp_2/1 -> tws_2/1, AndN/2
  BS_Req/3 -> cmp_3/1  "<testSig_PRV_ctOpnMax_DSM>"
  BS_Result/3 -> cmp_3/2  "<PRV_ctOpnMax_DSM>"
  cmp_3/1 -> tws_3/1, AndN/3
  BS_Req/4 -> cmp_4/1  "<testSig_PRV_tiOpnMax_DSM>"
  BS_Result/4 -> cmp_4/2  "<PRV_tiOpnMax_DSM>"
  cmp_4/1 -> tws_4/1, AndN/4
  BS_Req/5 -> cmp_5/1  "<testSig_PRV_ctPresShck_mp>"
  BS_Result/5 -> cmp_5/2  "<PRV_ctPresShck_mp>"
  cmp_5/1 -> tws_5/1, AndN/5
  BS_Req/6 -> cmp_6/1  "<testSig_PRVOpn_DSM>"
  BS_Result/6 -> cmp_6/2  "<PRVOpn_DSM>"
  cmp_6/1 -> tws_6/1, AndN/6
  BS_Req/7 -> cmp_7/1  "<testSig_PRV_st>"
  BS_Result/7 -> cmp_7/2  "<PRV_st>"
  cmp_7/1 -> tws_7/1, AndN/7
  BS_Req/8 -> cmp_8/1  "<testSig_PRVwearout_DSM>"
  BS_Result/8 -> cmp_8/2  "<PRVwearout_DSM>"
  cmp_8/1 -> tws_8/1, AndN/8
  BS_Req/9 -> cmp_9/1  "<testSig_PRV_stEvalRP>"
  BS_Result/9 -> cmp_9/2  "<PRV_stEvalRP>"
  cmp_9/1 -> tws_9/1, AndN/9
